simulink model "DinamicaCinematicaAtitude"  (R2023b)
settings: Solver=FixedStepAuto  StartTime=0.0  StopTime=tf  FixedStep=step_modelo  RelTol=1e-3
undefined symbols (not defined in the file or in its folder): AttKd_x, AttKd_y, AttKd_z, AttKp_x, AttKp_y, AttKp_z, man
settings Model: Creator=rodri  LastModifiedBy=rodri

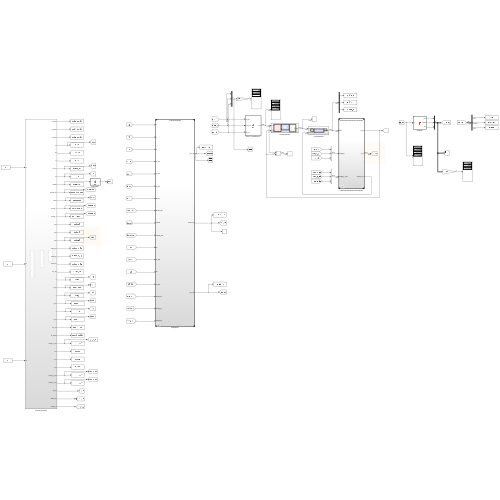
[thumbnail: Simulink's stored preview of the top-level diagram]
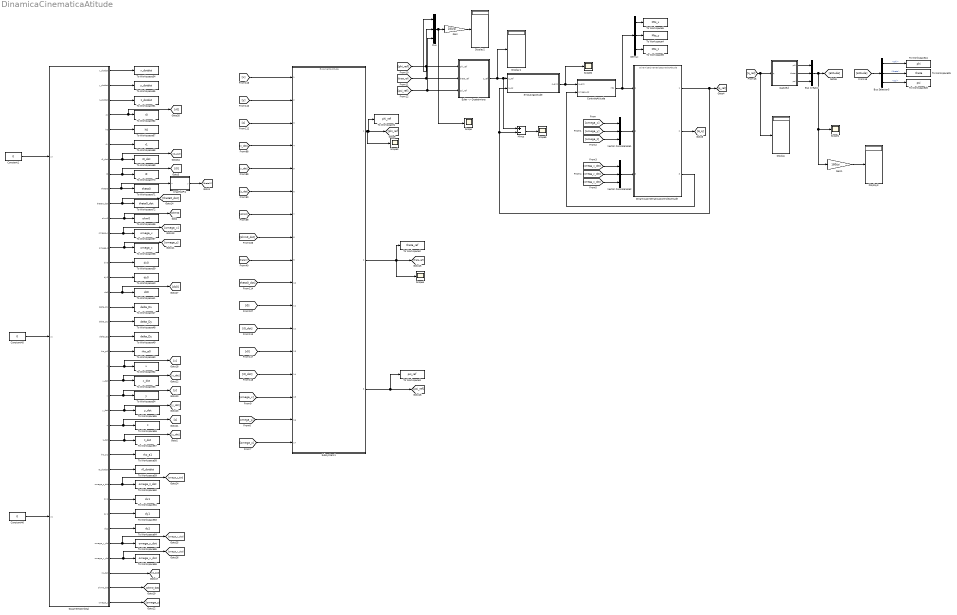
== system DinamicaCinematicaAtitude ==
  Bus Creator : BusCreator  Inputs=3
  Bus Selector5 : BusSelector  OutputSignals=phi,theta,psi
  Constant1 : Constant  Value=0
  Constant45 : Constant  Value=0
  Constant46 : Constant  Value=0
  ControleAtitude : Subsystem
  Demux : Demux  Outputs=3
  DinamicaCinematicaControleAtitude : ModelReference  ModelNameDialog=DinamicaCinematicaControleAtitude  ModelReferenceVersion=2.23
  Display{,1..3} (4 alike) : Display
  "Euler -> Quatérnions" : MATLAB Function  TreatAsAtomicUnit=on
  Gain : Gain  Gain=180/pi
  Gain1 : Gain  Gain=180/pi
  GuiamentoOrbital : Subsystem
  Minus : Sum  Inputs=+-
  Mux : Mux  Inputs=3
  Scope{,1..5} (6 alike) : Scope
  Subsystem1 : ModelReference  ModelNameDialog=GuiamentoAtitude  ModelReferenceVersion=2.6
  To Workspace1 : ToWorkspace  VariableName=phi_ref  SaveFormat=Timeseries  SampleTime=-1
  To Workspace2 : ToWorkspace  VariableName=theta_ref  SaveFormat=Timeseries  SampleTime=-1
  To Workspace24 : ToWorkspace  VariableName=phi  SaveFormat=Timeseries  SampleTime=-1
  To Workspace25 : ToWorkspace  VariableName=theta  SaveFormat=Timeseries  SampleTime=-1
  To Workspace26 : ToWorkspace  VariableName=psi  SaveFormat=Timeseries  SampleTime=-1
  To Workspace3 : ToWorkspace  VariableName=psi_ref  SaveFormat=Timeseries  SampleTime=-1
  To Workspace34 : ToWorkspace  VariableName=x_dotdot  SaveFormat=Timeseries  SampleTime=-1
  To Workspace35 : ToWorkspace  VariableName=y_dotdot  SaveFormat=Timeseries  SampleTime=-1
  To Workspace36 : ToWorkspace  VariableName=ohm0  SaveFormat=Timeseries  SampleTime=-1
  To Workspace37 : ToWorkspace  VariableName=omega_x  SaveFormat=Timeseries  SampleTime=-1
  To Workspace38 : ToWorkspace  VariableName=omega_z  SaveFormat=Timeseries  SampleTime=-1
  To Workspace39 : ToWorkspace  VariableName=dx0  SaveFormat=Timeseries  SampleTime=-1
  To Workspace4 : ToWorkspace  VariableName=Mts_y  SaveFormat=Timeseries  SampleTime=-1
  To Workspace40 : ToWorkspace  VariableName=dy0  SaveFormat=Timeseries  SampleTime=-1
  To Workspace41 : ToWorkspace  VariableName=dz0  SaveFormat=Timeseries  SampleTime=-1
  To Workspace47 : ToWorkspace  VariableName=delta_Dx  SaveFormat=Timeseries  SampleTime=-1
  To Workspace48 : ToWorkspace  VariableName=delta_Dy  SaveFormat=Timeseries  SampleTime=-1
  To Workspace49 : ToWorkspace  VariableName=delta_Dz  SaveFormat=Timeseries  SampleTime=-1
  To Workspace5 : ToWorkspace  VariableName=Mts_x  SaveFormat=Timeseries  SampleTime=-1
  To Workspace50 : ToWorkspace  VariableName=rho_a0  SaveFormat=Timeseries  SampleTime=-1
  To Workspace51 : ToWorkspace  VariableName=z_dotdot  SaveFormat=Timeseries  SampleTime=-1
  To Workspace52 : ToWorkspace  VariableName=x  SaveFormat=Timeseries  SampleTime=-1
  To Workspace53 : ToWorkspace  VariableName=x_dot  SaveFormat=Timeseries  SampleTime=-1
  To Workspace54 : ToWorkspace  VariableName=y  SaveFormat=Timeseries  SampleTime=-1
  To Workspace55 : ToWorkspace  VariableName=y_dot  SaveFormat=Timeseries  SampleTime=-1
  To Workspace56 : ToWorkspace  VariableName=z  SaveFormat=Timeseries  SampleTime=-1
  To Workspace57 : ToWorkspace  VariableName=z_dot  SaveFormat=Timeseries  SampleTime=-1
  To Workspace58 : ToWorkspace  VariableName=rho_a1  SaveFormat=Timeseries  SampleTime=-1
  To Workspace59 : ToWorkspace  VariableName=r0_dotdot  SaveFormat=Timeseries  SampleTime=-1
  To Workspace6 : ToWorkspace  VariableName=Mts_z  SaveFormat=Timeseries  SampleTime=-1
  To Workspace60 : ToWorkspace  VariableName=omega_z_dot  SaveFormat=Timeseries  SampleTime=-1
  To Workspace61 : ToWorkspace  VariableName=dx1  SaveFormat=Timeseries  SampleTime=-1
  To Workspace62 : ToWorkspace  VariableName=r0  SaveFormat=Timeseries  SampleTime=-1
  To Workspace63 : ToWorkspace  VariableName=dy1  SaveFormat=Timeseries  SampleTime=-1
  To Workspace64 : ToWorkspace  VariableName=dz1  SaveFormat=Timeseries  SampleTime=-1
  To Workspace65 : ToWorkspace  VariableName=omega_y_dot  SaveFormat=Timeseries  SampleTime=-1
  To Workspace66 : ToWorkspace  VariableName=omega_x_dot  SaveFormat=Timeseries  SampleTime=-1
  To Workspace67 : ToWorkspace  VariableName=h0  SaveFormat=Timeseries  SampleTime=-1
  To Workspace68 : ToWorkspace  VariableName=r1  SaveFormat=Timeseries  SampleTime=-1
  To Workspace69 : ToWorkspace  VariableName=r0_dot  SaveFormat=Timeseries  SampleTime=-1
  To Workspace70 : ToWorkspace  VariableName=i0  SaveFormat=Timeseries  SampleTime=-1
  To Workspace71 : ToWorkspace  VariableName=theta0  SaveFormat=Timeseries  SampleTime=-1
  To Workspace72 : ToWorkspace  VariableName=theta0_dot  SaveFormat=Timeseries  SampleTime=-1
  Vector Concatenate1 : Concatenate  NumInputs=3  Mode=Multidimensional array
  Vector Concatenate2 : Concatenate  NumInputs=3  Mode=Multidimensional array
  errosAngAtitude : Subsystem
  quat2eul : MATLAB Function  TreatAsAtomicUnit=on
  wrapTo2Pi1 : MATLAB Function  TreatAsAtomicUnit=on
  wires:
  GuiamentoOrbital/25(z) -> To Workspace56/1, [z]
  GuiamentoOrbital/16(dz0) -> [dz0], To Workspace41/1
  GuiamentoOrbital/10(theta0_dot) -> [theta0_dot], To Workspace72/1
  GuiamentoOrbital/15(dy0) -> To Workspace40/1
  GuiamentoOrbital/11(ohm0) -> [ohm0], To Workspace36/1
  GuiamentoOrbital/12(omega_x) -> To Workspace37/1, [omega_x]
  Constant1/1 -> GuiamentoOrbital/1(ux)
  GuiamentoOrbital/36(ohm0_dot) -> [ohm0_dot]
  GuiamentoOrbital/28(r0_dotdot) -> To Workspace59/1
  GuiamentoOrbital/13(omega_z) -> [omega_z], To Workspace38/1
  GuiamentoOrbital/37(omega_y) -> [omega_y]
  GuiamentoOrbital/20(rho_a0) -> To Workspace50/1
  GuiamentoOrbital/35(i0_dot) -> [i0_dot]
  Constant46/1 -> GuiamentoOrbital/3(uz)
  GuiamentoOrbital/34(omega_x_dot) -> [omega_x_dot], To Workspace66/1
  GuiamentoOrbital/27(rho_a1) -> To Workspace58/1
  GuiamentoOrbital/7(r0_dot) -> To Workspace69/1, [r0_dot]
  wrapTo2Pi1/1(y) -> [theta0]
  GuiamentoOrbital/9(theta0) -> To Workspace71/1, wrapTo2Pi1/1(u)
  GuiamentoOrbital/1(x_dotdot) -> To Workspace34/1
  GuiamentoOrbital/5(h0) -> To Workspace67/1
  GuiamentoOrbital/6(r1) -> To Workspace68/1
  GuiamentoOrbital/8(i0) -> [i0], To Workspace70/1
  GuiamentoOrbital/4(r0) -> To Workspace62/1, [r0]
  GuiamentoOrbital/21(x) -> To Workspace52/1, [x]
  GuiamentoOrbital/26(z_dot) -> [z_dot], To Workspace57/1
  GuiamentoOrbital/18(delta_Dy) -> To Workspace48/1
  GuiamentoOrbital/22(x_dot) -> To Workspace53/1, [x_dot]
  GuiamentoOrbital/23(y) -> To Workspace54/1, [y]
  Constant45/1 -> GuiamentoOrbital/2(uy)
  GuiamentoOrbital/24(y_dot) -> To Workspace55/1, [y_dot]
  GuiamentoOrbital/3(z_dotdot) -> To Workspace51/1
  GuiamentoOrbital/33(omega_y_dot) -> [omega_y_dot], To Workspace65/1
  GuiamentoOrbital/29(omega_z_dot) -> [omega_z_dot], To Workspace60/1
  GuiamentoOrbital/2(y_dotdot) -> To Workspace35/1
  GuiamentoOrbital/30(dx1) -> To Workspace61/1
  GuiamentoOrbital/32(dz1) -> To Workspace64/1
  GuiamentoOrbital/31(dy1) -> To Workspace63/1
  GuiamentoOrbital/19(delta_Dz) -> To Workspace49/1
  GuiamentoOrbital/14(dx0) -> To Workspace39/1
  GuiamentoOrbital/17(delta_Dx) -> To Workspace47/1
  Subsystem1/1 -> [phi_ref], To Workspace1/1, Scope3/1
  Subsystem1/3 -> To Workspace3/1, [psi_ref]
  Subsystem1/2 -> Scope4/1, [theta_ref], To Workspace2/1
  [omega_y] -> Vector Concatenate1/2
  [omega_z] -> Vector Concatenate1/3
  [omega_x_dot] -> Vector Concatenate2/1
  [omega_y_dot] -> Vector Concatenate2/2
  [omega_z_dot] -> Vector Concatenate2/3
  [omega_x] -> Vector Concatenate1/1
  DinamicaCinematicaControleAtitude/3 -> ControleAtitude/2(omega_rel)
  DinamicaCinematicaControleAtitude/1 -> [q_rel], Minus/2, errosAngAtitude/2(q_rel)
  [omega_z] -> Subsystem1/17
  [omega_y] -> Subsystem1/16
  [omega_x] -> Subsystem1/15
  [r0_dot] -> Subsystem1/14
  [r0] -> Subsystem1/13
  [i0] -> Subsystem1/11
  [i0_dot] -> Subsystem1/12
  [x] -> Subsystem1/1
  [y] -> Subsystem1/2
  [z] -> Subsystem1/3
  [x_dot] -> Subsystem1/4
  [y_dot] -> Subsystem1/5
  [z_dot] -> Subsystem1/6
  [ohm0] -> Subsystem1/7
  [ohm0_dot] -> Subsystem1/8
  [theta0] -> Subsystem1/9
  [theta0_dot] -> Subsystem1/10
  ControleAtitude/1(Mts) -> Demux/1, DinamicaCinematicaControleAtitude/1
  errosAngAtitude/1(q_erro) -> ControleAtitude/1(q_erro), Scope2/1
  [phi_ref] -> Mux/1, "Euler -> Quatérnions"/1(phi_ref)
  [theta_ref] -> "Euler -> Quatérnions"/2(theta_ref), Mux/2
  [psi_ref] -> "Euler -> Quatérnions"/3(psi_ref), Mux/3
  Vector Concatenate1/1 -> DinamicaCinematicaControleAtitude/2
  Vector Concatenate2/1 -> DinamicaCinematicaControleAtitude/3
  Bus Creator/1 -> Gain1/1, Scope1/1, [atitude]
  quat2eul/1(phi) -> Bus Creator/1
  quat2eul/3(psi) -> Bus Creator/3
  quat2eul/2(theta) -> Bus Creator/2
  Bus Selector5/2 -> To Workspace25/1  "<theta>"
  Bus Selector5/1 -> To Workspace24/1  "<phi>"
  Bus Selector5/3 -> To Workspace26/1  "<psi>"
  [atitude] -> Bus Selector5/1
  Demux/2 -> To Workspace4/1
  Demux/1 -> To Workspace5/1
  Demux/3 -> To Workspace6/1
  "Euler -> Quatérnions"/1(q_ref) -> Minus/1, errosAngAtitude/1(q_ref), Display1/1
  DinamicaCinematicaControleAtitude/2 -> [A_q]
  [q_rel] -> Display/1, quat2eul/1(q)
  Mux/1 -> Scope/1, Gain/1
  Gain/1 -> Display2/1
  Minus/1 -> Scope5/1
  Gain1/1 -> Display3/1

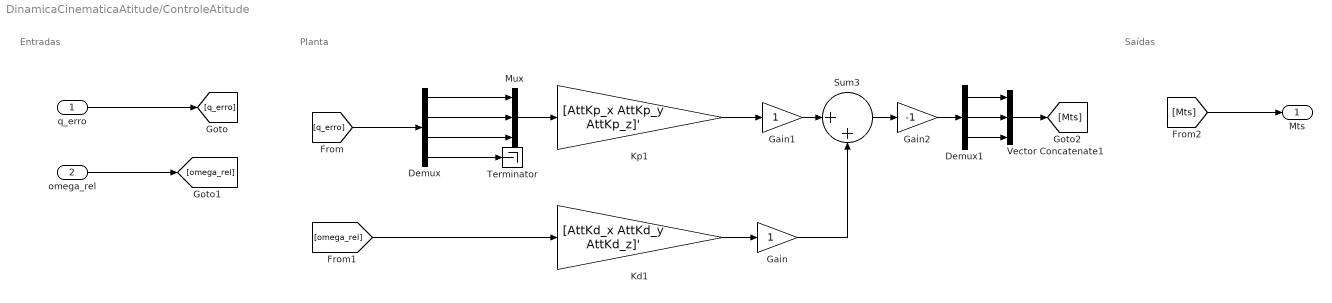
== system DinamicaCinematicaAtitude/ControleAtitude ==
  note: Entradas
  note: Planta
  note: Saídas
  q_erro : Inport
  omega_rel : Inport  Port=2
  Demux : Demux
  Demux1 : Demux  Outputs=3
  Gain : Gain
  Gain1 : Gain
  Gain2 : Gain  Gain=-1
  Kd1 : Gain  Gain=[AttKd_x AttKd_y AttKd_z]'
  Kp1 : Gain  Gain=[AttKp_x AttKp_y AttKp_z]'
  Mux : Mux  Inputs=3
  Sum3 : Sum  Inputs=|++
  Terminator : Terminator
  Vector Concatenate1 : Concatenate  NumInputs=3  Mode=Multidimensional array
  Mts : Outport
  wires:
  Kd1/1 -> Gain/1
  [q_erro] -> Demux/1
  Mux/1 -> Kp1/1
  Demux/1 -> Mux/1
  Demux/2 -> Mux/2
  Demux/3 -> Mux/3
  Demux/4 -> Terminator/1
  [omega_rel] -> Kd1/1
  Gain/1 -> Sum3/2
  Gain1/1 -> Sum3/1
  Kp1/1 -> Gain1/1
  Sum3/1 -> Gain2/1
  Demux1/1 -> Vector Concatenate1/1
  Demux1/2 -> Vector Concatenate1/2
  Demux1/3 -> Vector Concatenate1/3
  Vector Concatenate1/1 -> [Mts]
  q_erro/1 -> [q_erro]
  omega_rel/1 -> [omega_rel]
  [Mts] -> Mts/1
  Gain2/1 -> Demux1/1

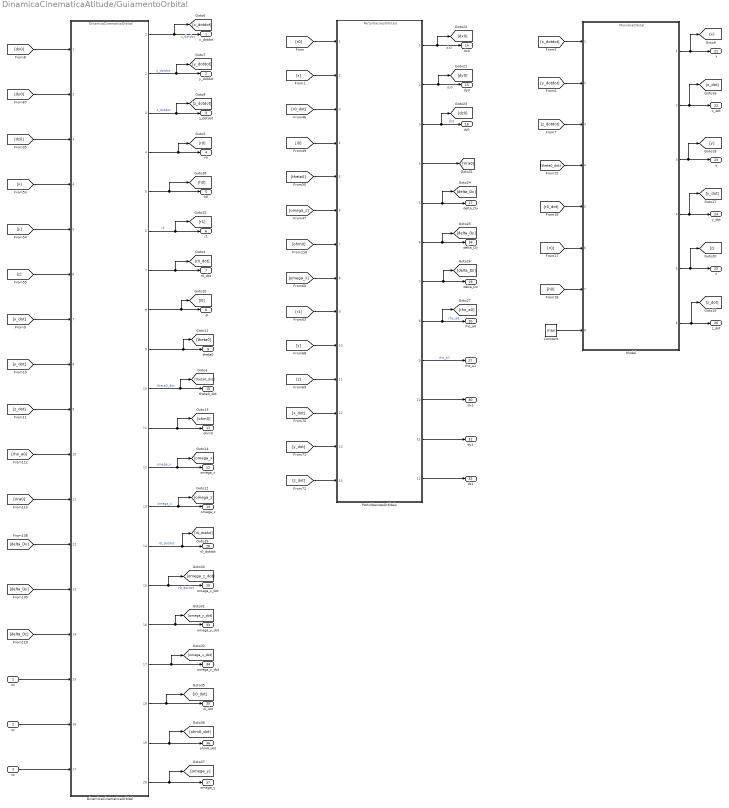
== system DinamicaCinematicaAtitude/GuiamentoOrbital ==
  ux : Inport  OutDataTypeStr=double  PortDimensions=1
  uy : Inport  Port=2  OutDataTypeStr=double  PortDimensions=1
  uz : Inport  Port=3  OutDataTypeStr=double  PortDimensions=1
  Constant : Constant  Value=man
  DinamicaCinematicaOrbital : ModelReference  ModelNameDialog=DinamicaCinematicaOrbital  ModelReferenceVersion=4.0
  Model : ModelReference  ModelNameDialog=ManobraOrbital.slx  ModelReferenceVersion=4.2
  PerturbacoesOrbitais : ModelReference  ModelNameDialog=PerturbacoesOrbitais  ModelReferenceVersion=4.0
  x_dotdot : Outport  OutDataTypeStr=double  PortDimensions=1  SampleTime=0
  y_dotdot : Outport  Port=2  OutDataTypeStr=double  PortDimensions=1  SampleTime=0
  z_dotdot : Outport  Port=3  OutDataTypeStr=double  PortDimensions=1  SampleTime=0
  r0 : Outport  Port=4  OutDataTypeStr=double  PortDimensions=1  SampleTime=0
  h0 : Outport  Port=5  OutDataTypeStr=double  PortDimensions=1  SampleTime=0
  r1 : Outport  Port=6  OutDataTypeStr=double  PortDimensions=1  SampleTime=0
  r0_dot : Outport  Port=7  OutDataTypeStr=double  PortDimensions=1  SampleTime=0
  i0 : Outport  Port=8  OutDataTypeStr=double  PortDimensions=1  SampleTime=0
  theta0 : Outport  Port=9  OutDataTypeStr=double  PortDimensions=1  SampleTime=0
  theta0_dot : Outport  Port=10  OutDataTypeStr=double  PortDimensions=1  SampleTime=0
  ohm0 : Outport  Port=11  OutDataTypeStr=double  PortDimensions=1  SampleTime=0
  omega_x : Outport  Port=12  OutDataTypeStr=double  PortDimensions=1  SampleTime=0
  omega_z : Outport  Port=13  OutDataTypeStr=double  PortDimensions=1  SampleTime=0
  dx0 : Outport  Port=14  OutDataTypeStr=double  PortDimensions=1  SampleTime=[1,0]
  dy0 : Outport  Port=15  OutDataTypeStr=double  PortDimensions=1  SampleTime=[1,0]
  dz0 : Outport  Port=16  OutDataTypeStr=double  PortDimensions=1  SampleTime=[1,0]
  delta_Dx : Outport  Port=17  OutDataTypeStr=double  PortDimensions=1  SampleTime=[1,0]
  delta_Dy : Outport  Port=18  OutDataTypeStr=double  PortDimensions=1  SampleTime=[1,0]
  delta_Dz : Outport  Port=19  OutDataTypeStr=double  PortDimensions=1  SampleTime=[1,0]
  rho_a0 : Outport  Port=20  OutDataTypeStr=double  PortDimensions=1  SampleTime=[1,0]
  x : Outport  Port=21  OutDataTypeStr=double  PortDimensions=1  SampleTime=0
  x_dot : Outport  Port=22  OutDataTypeStr=double  PortDimensions=1  SampleTime=0
  y : Outport  Port=23  OutDataTypeStr=double  PortDimensions=1  SampleTime=0
  y_dot : Outport  Port=24  OutDataTypeStr=double  PortDimensions=1  SampleTime=0
  z : Outport  Port=25  OutDataTypeStr=double  PortDimensions=1  SampleTime=0
  z_dot : Outport  Port=26  OutDataTypeStr=double  PortDimensions=1  SampleTime=0
  rho_a1 : Outport  Port=27  OutDataTypeStr=double  PortDimensions=1  SampleTime=[1,0]
  r0_dotdot : Outport  Port=28  OutDataTypeStr=double  PortDimensions=1  SampleTime=0
  omega_z_dot : Outport  Port=29  OutDataTypeStr=double  PortDimensions=1  SampleTime=0
  dx1 : Outport  Port=30  OutDataTypeStr=double  PortDimensions=1  SampleTime=[1,0]
  dy1 : Outport  Port=31  OutDataTypeStr=double  PortDimensions=1  SampleTime=[1,0]
  dz1 : Outport  Port=32  OutDataTypeStr=double  PortDimensions=1  SampleTime=[1,0]
  omega_y_dot : Outport  Port=33  OutDataTypeStr=double  PortDimensions=1  SampleTime=0
  omega_x_dot : Outport  Port=34  OutDataTypeStr=double  PortDimensions=1  SampleTime=0
  i0_dot : Outport  Port=35  OutDataTypeStr=double  PortDimensions=1  SampleTime=0
  ohm0_dot : Outport  Port=36  OutDataTypeStr=double  PortDimensions=1  SampleTime=0
  omega_y : Outport  Port=37  OutDataTypeStr=double  PortDimensions=1  SampleTime=0
  wires:
  DinamicaCinematicaOrbital/6 -> r1/1, [r1]  "r1"
  PerturbacoesOrbitais/4 -> [Vra0]
  DinamicaCinematicaOrbital/8 -> i0/1, [i0]
  DinamicaCinematicaOrbital/12 -> omega_x/1, [omega_x]  "omega_x"
  DinamicaCinematicaOrbital/10 -> theta0_dot/1, [theta0_dot]  "theta0_dot"
  PerturbacoesOrbitais/9 -> rho_a1/1  "rho_a1"
  PerturbacoesOrbitais/7 -> delta_Dz/1, [delta_Dz]
  DinamicaCinematicaOrbital/1 -> x_dotdot/1, [x_dotdot]  "x_dotdot"
  PerturbacoesOrbitais/2 -> [dy0], dy0/1  "dy0"
  DinamicaCinematicaOrbital/9 -> theta0/1, [theta0]
  PerturbacoesOrbitais/6 -> delta_Dy/1, [delta_Dy]
  PerturbacoesOrbitais/1 -> dx0/1, [dx0]  "dx0"
  Model/5 -> z/1, [z]
  Model/4 -> y_dot/1, [y_dot]
  Model/1 -> x/1, [x]
  Model/3 -> [y], y/1
  PerturbacoesOrbitais/3 -> dz0/1, [dz0]  "dz0"
  DinamicaCinematicaOrbital/7 -> r0_dot/1, [r0_dot]
  PerturbacoesOrbitais/8 -> [rho_a0], rho_a0/1  "rho_a0"
  DinamicaCinematicaOrbital/5 -> h0/1, [h0]
  DinamicaCinematicaOrbital/13 -> omega_z/1, [omega_z]  "omega_z"
  DinamicaCinematicaOrbital/3 -> z_dotdot/1, [z_dotdot]  "z_dotdot"
  DinamicaCinematicaOrbital/2 -> y_dotdot/1, [y_dotdot]  "y_dotdot"
  DinamicaCinematicaOrbital/4 -> r0/1, [r0]
  Model/6 -> z_dot/1, [z_dot]
  DinamicaCinematicaOrbital/11 -> ohm0/1, [ohm0]
  PerturbacoesOrbitais/5 -> delta_Dx/1, [delta_Dx]
  Model/2 -> x_dot/1, [x_dot]
  DinamicaCinematicaOrbital/14 -> r0_dotdot/1, [r0_dotdot]  "r0_dotdot"
  DinamicaCinematicaOrbital/15 -> omega_z_dot/1, [omega_z_dot]  "r0_dotdot"
  PerturbacoesOrbitais/10 -> dx1/1
  PerturbacoesOrbitais/11 -> dy1/1
  PerturbacoesOrbitais/12 -> dz1/1
  DinamicaCinematicaOrbital/16 -> omega_y_dot/1, [omega_y_dot]
  DinamicaCinematicaOrbital/17 -> omega_x_dot/1, [omega_x_dot]
  DinamicaCinematicaOrbital/18 -> i0_dot/1, [i0_dot]
  DinamicaCinematicaOrbital/19 -> [ohm0_dot], ohm0_dot/1
  DinamicaCinematicaOrbital/20 -> [omega_y], omega_y/1
  [dx0] -> DinamicaCinematicaOrbital/1
  [dy0] -> DinamicaCinematicaOrbital/2
  [dz0] -> DinamicaCinematicaOrbital/3
  [x] -> DinamicaCinematicaOrbital/4
  [y] -> DinamicaCinematicaOrbital/5
  [z] -> DinamicaCinematicaOrbital/6
  [x_dot] -> DinamicaCinematicaOrbital/7
  [y_dot] -> DinamicaCinematicaOrbital/8
  [z_dot] -> DinamicaCinematicaOrbital/9
  [Vra0] -> DinamicaCinematicaOrbital/11
  [rho_a0] -> DinamicaCinematicaOrbital/10
  [delta_Dx] -> DinamicaCinematicaOrbital/12
  [delta_Dy] -> DinamicaCinematicaOrbital/13
  [delta_Dz] -> DinamicaCinematicaOrbital/14
  ux/1 -> DinamicaCinematicaOrbital/15
  uy/1 -> DinamicaCinematicaOrbital/16
  uz/1 -> DinamicaCinematicaOrbital/17
  [r0] -> PerturbacoesOrbitais/1
  [x] -> PerturbacoesOrbitais/2
  [r0_dot] -> PerturbacoesOrbitais/3
  [i0] -> PerturbacoesOrbitais/4
  [theta0] -> PerturbacoesOrbitais/5
  [omega_z] -> PerturbacoesOrbitais/6
  [ohm0] -> PerturbacoesOrbitais/7
  [omega_x] -> PerturbacoesOrbitais/8
  [r1] -> PerturbacoesOrbitais/9
  [y] -> PerturbacoesOrbitais/10
  [z] -> PerturbacoesOrbitais/11
  [x_dot] -> PerturbacoesOrbitais/12
  [y_dot] -> PerturbacoesOrbitais/13
  [z_dot] -> PerturbacoesOrbitais/14
  [x_dotdot] -> Model/1
  [y_dotdot] -> Model/2
  [z_dotdot] -> Model/3
  [theta0_dot] -> Model/4
  [r0_dot] -> Model/5
  [r0] -> Model/6
  [h0] -> Model/7
  Constant/1 -> Model/8

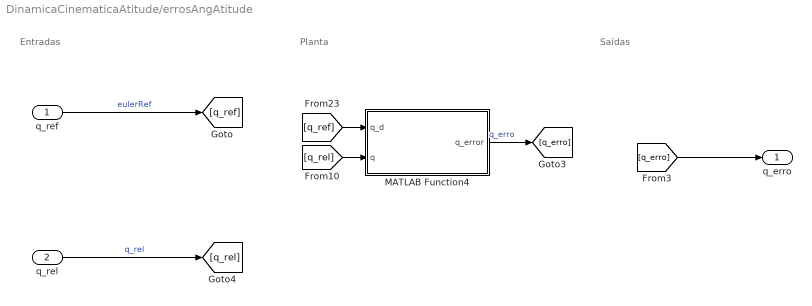
== system DinamicaCinematicaAtitude/errosAngAtitude ==
  note: Planta
  note: Saídas
  note: Entradas
  q_ref : Inport
  q_rel : Inport  Port=2
  MATLAB Function4 : MATLAB Function  TreatAsAtomicUnit=on
  q_erro : Outport
  wires:
  [q_ref] -> MATLAB Function4/1(q_d)
  [q_rel] -> MATLAB Function4/2(q)
  MATLAB Function4/1(q_error) -> [q_erro]  "q_erro"
  [q_erro] -> q_erro/1
  q_rel/1 -> [q_rel]  "q_rel"
  q_ref/1 -> [q_ref]  "eulerRef"

== matlab function DinamicaCinematicaAtitude/quat2eul ==
  data: q input; phi output; theta output; psi output
function [phi,theta,psi] = fcn(q)

euler = quat2eul([q(1) q(2) q(3) q(4)]);

phi = euler(1);
theta = euler(2);
psi = euler(3);


% q1 = q(1);
% q2 = q(2);
% q3 = q(3);
% q4 = q(4);
% 
% y = [atan2((2*q2*q4+2*q1*q3),(-2*q3*q4+2*q1*q2))
%     acos(min(1, max(-1, (q4^2-q3^2-q2^2+q1^2))));
%     atan2((2*q2*q4-2*q1*q3),(2*q3*q4+2*q1*q2))];
% 
% phi = y(1);
% theta = y(2);
% psi = y(3);


% 
% Quando theta está no primeiro e segundo quadrante -> usar if.
% Quando theta está no terceiro e quarto quadrando -> usar else.
% 
% if cond>0
%     euler = [atan2(2*(q1*q3+q0*q2),2*(-q2*q3+q0*q1))
%         acos(q3^2-q2^2-q1^2+q0^2)
%         atan2(2*(q1*q3-q0*q2),2*(q2*q3+q0*q1))];
% else
%     euler = [atan2(-2*(q1*q3+q0*q2),-2*(-q2*q3+q0*q1))
%         -acos(q3^2-q2^2-q1^2+q0^2)
%         atan2(-2*(q1*q3-q0*q2),-2*(q2*q3+q0*q1))];
% end

== matlab function DinamicaCinematicaAtitude/Euler -> Quatérnions ==
  data: phi_ref input; q_ref output; theta_ref input; psi_ref input
function q_ref = fcn(phi_ref,theta_ref,psi_ref)

phi = phi_ref;
theta = theta_ref;
psi = psi_ref;

q_ref = eul2quat([phi theta psi]);

%tol = 0.0001;
% q_ref = [cos(psi/2)*cos(theta/2)*cos(phi/2) - sin(psi/2)*cos(theta/2)*sin(phi/2)
%     cos(psi/2)*cos(phi/2)*sin(theta/2) + sin(psi/2)*sin(theta/2)*sin(phi/2)
%     cos(psi/2)*sin(theta/2)*sin(phi/2) - sin(psi/2)*cos(phi/2)*sin(theta/2)
%     cos(psi/2)*cos(theta/2)*sin(phi/2) + cos(theta/2)*cos(phi/2)*sin(psi/2)];
% 
% if q_ref(1)>=-tol && q_ref(1) <= tol
%     q_ref(1) = 0;
%     q_ref(2) = 0;
%     q_ref(3) = 0;
%     q_ref(4) = 0;
% end

== matlab function DinamicaCinematicaAtitude/errosAngAtitude/MATLAB Function4 ==
  data: q_d input; q_error output; q input
function q_error = fcn(q_d,q)

qt1 = q_d(1);
qt2 = q_d(2);
qt3 = q_d(3);
qt4 = q_d(4);

qs1 = q(1);
qs2 = q(2);
qs3 = q(3);
qs4 = q(4);

q_error = [qt4 qt3 -qt2 -qt1
    -qt3 qt4 qt1 -qt2
    qt2 -qt1 qt4 -qt3
    qt1 qt2 qt3 qt4]*[qs1;qs2;qs3;qs4];

== matlab function DinamicaCinematicaAtitude/wrapTo2Pi1 ==
  data: u input; y output
function y = fcn(u)



y = wrapTo2Pi(u);
